simulink model "HBF"  (R2024b)
settings: Solver=VariableStepAuto  StartTime=0.0  StopTime=10.0  RelTol=1e-3
libraries: dspfdesign x3
settings Model: Creator=gjp88  LastModifiedBy=gjp88

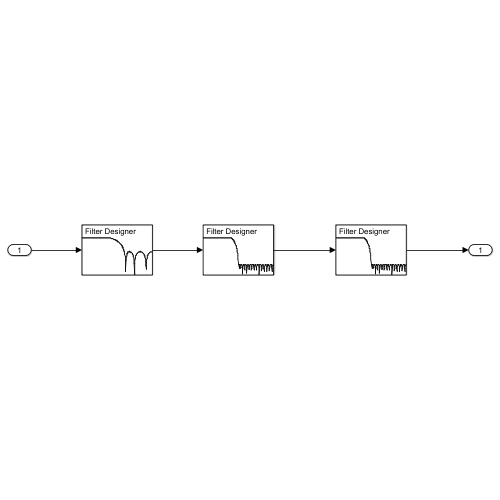
[thumbnail: Simulink's stored preview of the top-level diagram]
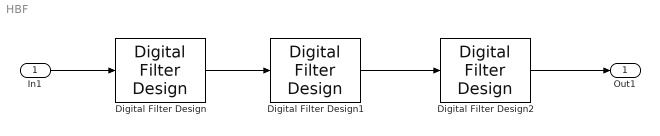
== system HBF ==
  In1 : Inport
  Digital Filter Design : dspfdesign/Digital Filter Design  mwdsp_browser_bugfix_var=off
  Digital Filter Design1 : dspfdesign/Digital Filter Design  mwdsp_browser_bugfix_var=off
  Digital Filter Design2 : dspfdesign/Digital Filter Design  mwdsp_browser_bugfix_var=off
  Out1 : Outport
  wires:
  Digital Filter Design/1 -> Digital Filter Design1/1
  Digital Filter Design1/1 -> Digital Filter Design2/1
  In1/1 -> Digital Filter Design/1
  Digital Filter Design2/1 -> Out1/1
